simulink model "PCS_3Phase_Grid_Manual"  (R2025a)
settings: Solver=ode4  StartTime=0.0  StopTime=0.5  FixedStep=1e-5  RelTol=1e-3
InitFcn:
  | v = str2double(get_param('PCS_3Phase_Grid_Manual/Vpcs_set', 'Value'));p = str2double(get_param('PCS_3Phase_Grid_Manual/Phase_set', 'Value'));set_param('PCS_3Phase_Grid_Manual/PCS', 'Voltage', num2str(v));set_param('PCS_3Phase_Grid_Manual/PCS', 'PhaseAngle', num2str(p));
libraries: spsThreePhaseSourceLib x2, spsThreePhaseSeriesRLCBranchLib x1, spsThreePhaseVIMeasurementLib x1, spspowerguiLib x1
Description:
  | Three-Phase PCS Simulation (native sps blocks)
  | R=0.1Ohm, L=5.0mH
  | P_total, Q_total = CONSTANT (no 100Hz ripple)
settings Model: Creator=jicai  LastModifiedBy=jicai

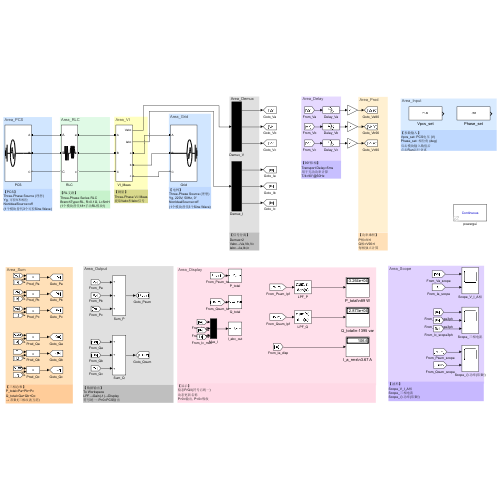
[thumbnail: Simulink's stored preview of the top-level diagram]
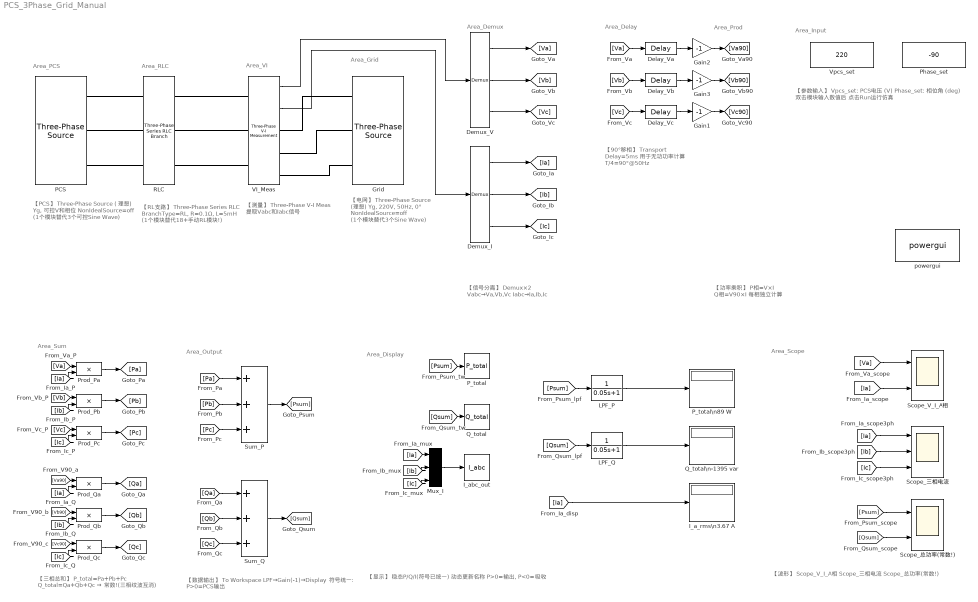
== system PCS_3Phase_Grid_Manual ==
  note: Area_Grid
  note: Area_VI
  note: Area_RLC
  note: Area_PCS
  note: Area_Demux
  note: Area_Delay
  note: Area_Prod
  note: Area_Sum
  note: Area_Output
  note: Area_Display
  note: Area_Scope
  note: 【电网】
      | Three-Phase Source (理想)
      | Yg, 220V, 50Hz, 0°
      | NonIdealSource=off
      | (1个模块替代3个Sine Wave)
  note: 【测量】
      | Three-Phase V-I Meas
      | 提取Vabc和Iabc信号
  note: 【RL支路】
      | Three-Phase Series RLC
      | BranchType=RL, R=0.1Ω, L=5mH
      | (1个模块替代18+手动RL模块!)
  note: 【PCS】
      | Three-Phase Source (理想)
      | Yg, 可控V和相位
      | NonIdealSource=off
      | (1个模块替代3个可控Sine Wave)
  note: 【信号分离】
      | Demux×2
      | Vabc→Va,Vb,Vc
      | Iabc→Ia,Ib,Ic
  note: 【90°移相】
      | Transport Delay=5ms
      | 用于无功功率计算
      | T/4=90°@50Hz
  note: 【功率乘积】
      | P相=V×I
      | Q相=V90×I
      | 每相独立计算
  note: 【三相总和】
      | P_total=Pa+Pb+Pc
      | Q_total=Qa+Qb+Qc
      | → 常数!(三相纹波互消)
  note: 【数据输出】
      | To Workspace
      | LPF→Gain(-1)→Display
      | 符号统一: P>0=PCS输出
  note: 【显示】
      | 稳态P/Q/I(符号已统一)
      | 动态更新名称
      | P>0=输出, P<0=吸收
  note: 【波形】
      | Scope_V_I_A相
      | Scope_三相电流
      | Scope_总功率(常数!)
  note: Area_Input
  note: 【参数输入】
      | Vpcs_set: PCS电压 (V)
      | Phase_set: 相位角 (deg)
      | 双击模块输入数值后
      | 点击Run运行仿真
  Delay_Va : TransportDelay  DelayTime=0.005
  Delay_Vb : TransportDelay  DelayTime=0.005
  Delay_Vc : TransportDelay  DelayTime=0.005
  Demux_I : Demux  Outputs=3
  Demux_V : Demux  Outputs=3
  Gain1 : Gain  Gain=-1
  Gain2 : Gain  Gain=-1
  Gain3 : Gain  Gain=-1
  Grid : spsThreePhaseSourceLib/Three-Phase Source  InternalConnection=Yg  VoltagePhases=off  Voltage=220  PhaseAngle=0  Voltage_phases=[25e3 25e3 25e3]/sqrt(3)  PhaseAngles_phases=[0 -120 +120]  Frequency=50  NonIdealSource=off  SpecifyImpedance=off  Resistance=0.8929  Inductance=16.58e-3  ShortCircuitLevel=100e6  BaseVoltage=25e3  XRratio=7  BusType=swing  Pref=10e3  Qref=0  Prefabc=[10e3, 10e3, 10e3]  Qrefabc=[0, 0, 0]  Qmin=-inf  Qmax=inf
  I_a_rms\n3.67 A : Display
  I_abc_out : ToWorkspace  VariableName=I_abc  SampleTime=-1
  LPF_P : TransferFcn  Denominator=[0.05 1]
  LPF_Q : TransferFcn  Denominator=[0.05 1]
  Mux_I : Mux  Inputs=3
  PCS : spsThreePhaseSourceLib/Three-Phase Source  InternalConnection=Yg  VoltagePhases=off  Voltage=220  PhaseAngle=-90  Voltage_phases=[25e3 25e3 25e3]/sqrt(3)  PhaseAngles_phases=[0 -120 +120]  Frequency=50  NonIdealSource=off  SpecifyImpedance=off  Resistance=0.8929  Inductance=16.58e-3  ShortCircuitLevel=100e6  BaseVoltage=25e3  XRratio=7  BusType=swing  Pref=10e3  Qref=0  Prefabc=[10e3, 10e3, 10e3]  Qrefabc=[0, 0, 0]  Qmin=-inf  Qmax=inf
  P_total : ToWorkspace  VariableName=P_total  SampleTime=-1
  P_total\n89 W : Display
  Phase_set : Constant  Value=-90
  Prod_Pa : Product  Inputs=**
  Prod_Pb : Product  Inputs=**
  Prod_Pc : Product  Inputs=**
  Prod_Qa : Product  Inputs=**
  Prod_Qb : Product  Inputs=**
  Prod_Qc : Product  Inputs=**
  Q_total : ToWorkspace  VariableName=Q_total  SampleTime=-1
  Q_total\n-1395 var : Display
  RLC : spsThreePhaseSeriesRLCBranchLib/Three-Phase Series RLC Branch  LConnTagsString=A|B|C  RConnTagsString=A|B|C  BranchType=RL  Resistance=0.1  Inductance=0.005  Capacitance=1e-6  Measurements=None
  Scope_V_I_A相 : Scope  NumInputPorts=2
  Scope_三相电流 : Scope  NumInputPorts=3
  Scope_总功率(常数!) : Scope  NumInputPorts=2
      settings: ActiveDisplayYMinimum=-3183.9654567396947  ActiveDisplayYMaximum=43915.49482311411
  Sum_P : Sum  Inputs=+++
  Sum_Q : Sum  Inputs=+++
  VI_Meas : spsThreePhaseVIMeasurementLib/Three-Phase V-I Measurement  VoltageMeasurement=phase-to-ground  SetLabelV=off  LabelV=Vabc  Vpu=off  VpuLL=off  CurrentMeasurement=yes  SetLabelI=off  LabelI=Iabc  Ipu=off  Pbase=100e6  Vbase=500e3  OutputType=Complex  PhasorSimulation=off  PSBequivalent=0
  Vpcs_set : Constant  Value=220
  powergui : spspowerguiLib/powergui  Priority=1  SimulationMode=Continuous  SampleTime=50e-6  frequency=60  Iterations=50  frequencyindice=50  Pbase=100e6  ErrMax=1e-4  UnitsV=kV  UnitsW=MW  buscounter=0  FunctionMessages=off  echomessages=off  EnableUseOfTLC=off  CurrentSourceSwitches=off  DisableSnubberDevices=off  DisableRonSwitches=off  DisableVfSwitches=off  DisplayEquations=off  AutomaticDiscreteSolvers=off  SolverType=Tustin/Backward Euler (TBE)  Interpol=off  ExternalGateDelay=off  methode=off  Ts=100  x0status=blocks  SPID=on  SwTol=0  HookPort=off  NonlinearTolerance=1e-4  nMaxIteration=100  ContinueOnMaxIteration=off  RestoreLinks=warning  ResistiveCurrentMeasurement=off  Frange=[0:2:500]  Ylog=off  Xlog=on  ShowGrid=off  save=off  variable=ZData  structure=0  ZoomFFT=off  StartTime=0.0  cycles=1  DisplayStyle=1  fundamental=60  FreqAxis=off  MaxFrequency=1000  frequencyindicesteady=1  RmsSteady=1  display=off
  wires:
  VI_Meas/1 -> Demux_V/1
  VI_Meas/2 -> Demux_I/1
  Demux_V/1 -> [Va]
  Demux_V/2 -> [Vb]
  Demux_V/3 -> [Vc]
  Demux_I/1 -> [Ia]
  Demux_I/2 -> [Ib]
  Demux_I/3 -> [Ic]
  [Va] -> Delay_Va/1
  Delay_Va/1 -> Gain2/1
  [Vb] -> Delay_Vb/1
  Delay_Vb/1 -> Gain3/1
  [Vc] -> Delay_Vc/1
  Delay_Vc/1 -> Gain1/1
  [Va] -> Prod_Pa/1
  [Ia] -> Prod_Pa/2
  [Va90] -> Prod_Qa/1
  [Ia] -> Prod_Qa/2
  Prod_Pa/1 -> [Pa]
  Prod_Qa/1 -> [Qa]
  [Vb] -> Prod_Pb/1
  [Ib] -> Prod_Pb/2
  [Vb90] -> Prod_Qb/1
  [Ib] -> Prod_Qb/2
  Prod_Pb/1 -> [Pb]
  Prod_Qb/1 -> [Qb]
  [Vc] -> Prod_Pc/1
  [Ic] -> Prod_Pc/2
  [Vc90] -> Prod_Qc/1
  [Ic] -> Prod_Qc/2
  Prod_Pc/1 -> [Pc]
  Prod_Qc/1 -> [Qc]
  [Pa] -> Sum_P/1
  [Qa] -> Sum_Q/1
  [Pb] -> Sum_P/2
  [Qb] -> Sum_Q/2
  [Pc] -> Sum_P/3
  [Qc] -> Sum_Q/3
  Sum_P/1 -> [Psum]
  Sum_Q/1 -> [Qsum]
  [Psum] -> P_total/1
  [Qsum] -> Q_total/1
  [Ia] -> Mux_I/1
  [Ib] -> Mux_I/2
  [Ic] -> Mux_I/3
  Mux_I/1 -> I_abc_out/1
  [Psum] -> LPF_P/1
  [Qsum] -> LPF_Q/1
  LPF_P/1 -> P_total\n89 W/1
  [Ia] -> I_a_rms\n3.67 A/1
  [Va] -> Scope_V_I_A相/1
  [Ia] -> Scope_V_I_A相/2
  [Ia] -> Scope_三相电流/1
  [Ib] -> Scope_三相电流/2
  [Ic] -> Scope_三相电流/3
  [Psum] -> Scope_总功率(常数!)/1
  [Qsum] -> Scope_总功率(常数!)/2
  LPF_Q/1 -> Q_total\n-1395 var/1
  Gain2/1 -> [Va90]
  Gain3/1 -> [Vb90]
  Gain1/1 -> [Vc90]
  connections:
  VI_Meas/RConn1 -- Grid/RConn1
  VI_Meas/RConn2 -- Grid/RConn2
  VI_Meas/RConn3 -- Grid/RConn3
  RLC/LConn1 -- PCS/RConn1
  RLC/LConn2 -- PCS/RConn2
  RLC/LConn3 -- PCS/RConn3
  RLC/RConn1 -- VI_Meas/LConn1
  RLC/RConn2 -- VI_Meas/LConn2
  RLC/RConn3 -- VI_Meas/LConn3
